simulink model "rwnn_pid_pso"  (R2021a)
settings: Solver=VariableStepAuto  StartTime=0.0  StopTime=10.0  RelTol=1e-3
PreLoadFcn:
  | b1=1
  | b2=1
  | b3=1
  | b4=1
  | a1=1
  | a2=1
  | a3=1
  | a4=1
  | qq1=1
  | qq2=1
  | qq3=1
  | qq4=1
  | w1=1
  | w2=1
  | w3=1
  | w4=1
  | ql=1
libraries: pid_lib x1
settings Model: Creator=mynam  LastModifiedBy=mynam

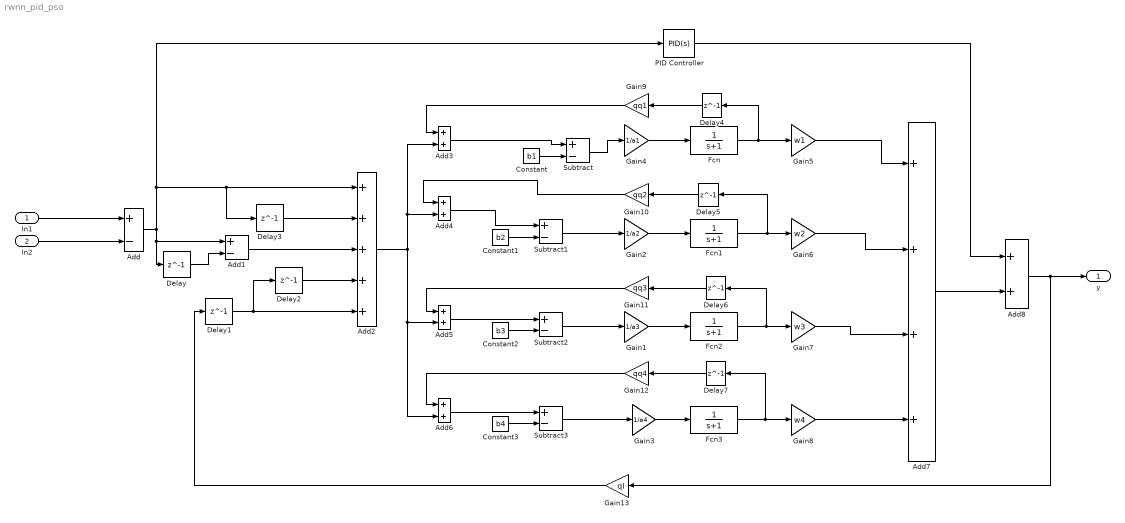
== system rwnn_pid_pso ==
  In1 : Inport
  In2 : Inport  Port=2
   Fcn{,1..3} (4 alike) : TransferFcn  Denominator=[1 1]
  Add : Sum  Inputs=+-
  Add1 : Sum  Inputs=+-
  Add2 : Sum  Inputs=+++++
  Add{3..6,8} (5 alike) : Sum
  Add7 : Sum  Inputs=++++
  Constant : Constant  Value=b1
  Constant1 : Constant  Value=b2
  Constant2 : Constant  Value=b3
  Constant3 : Constant  Value=b4
  Delay{,1..7} (8 alike) : Delay  DelayLength=1
  Gain1 : Gain  Gain=1/a3
  Gain10 : Gain  Gain=qq2
  Gain11 : Gain  Gain=qq3
  Gain12 : Gain  Gain=qq4
  Gain13 : Gain  Gain=ql
  Gain2 : Gain  Gain=1/a2
  Gain3 : Gain  Gain=1/a4
  Gain4 : Gain  Gain=1/a1
  Gain5 : Gain  Gain=w1
  Gain6 : Gain  Gain=w2
  Gain7 : Gain  Gain=w3
  Gain8 : Gain  Gain=w4
  Gain9 : Gain  Gain=qq1
  PID Controller : pid_lib/PID Controller  Controller=PID  Form=Parallel  TimeDomain=Continuous-time  UseExternalTs=off  SampleTime=-1  IntegratorMethod=Forward Euler  FilterMethod=Forward Euler  ControllerParametersSource=internal  P=1  I=1  D=0  UseFilter=on  N=100  TunerSelectOption=Transfer Function Based (PID Tuner App)  InitialConditionSource=internal  InitialConditionForIntegrator=0  InitialConditionForFilter=0  DifferentiatorICPrevScaledInput=0  ExternalReset=none  TrackingMode=off  Kt=1  LimitOutput=off  SatLimitsSource=internal  UpperSaturationLimit=inf  LowerSaturationLimit=-inf  LinearizeAsGain=on  AntiWindupMode=none  Kb=1  POutMin=[]  POutMax=[]  IOutMin=[]  IOutMax=[]  DOutMin=[]  DOutMax=[]  NOutMin=[]  NOutMax=[]  SumOutMin=[]  SumOutMax=[]  SaturationOutMin=[]  SaturationOutMax=[]  PParamMin=[]  PParamMax=[]  IParamMin=[]  IParamMax=[]  DParamMin=[]  DParamMax=[]  NParamMin=[]  NParamMax=[]  KbParamMin=[]  KbParamMax=[]  KtParamMin=[]  KtParamMax=[]  KbOutMin=[]  KbOutMax=[]  KtOutMin=[]  KtOutMax=[]  IntegratorOutMin=[]  IntegratorOutMax=[]  FilterOutMin=[]  FilterOutMax=[]  SumI1OutMin=[]  SumI1OutMax=[]  SumI2OutMin=[]  SumI2OutMax=[]  SumI3OutMin=[]  SumI3OutMax=[]  SumI4OutMin=[]  SumI4OutMax=[]  SumDOutMin=[]  SumDOutMax=[]  DifferentiatorOutMin=[]  DifferentiatorOutMax=[]  FilterDiffOutCoefMin=[]  FilterDiffOutCoefMax=[]  ReciprocalOutMin=[]  ReciprocalOutMax=[]  SumDenOutMin=[]  SumDenOutMax=[]  SumNumOutMin=[]  SumNumOutMax=[]  DivideOutMin=[]  DivideOutMax=[]  UdiffTsProdOutMin=[]  UdiffTsProdOutMax=[]  NTsProdOutMin=[]  NTsProdOutMax=[]  UintegralTsProdOutMin=[]  UintegralTsProdOutMax=[]  UngainTsProdOutMin=[]  UngainTsProdOutMax=[]  IntegratorContinuousStateAttributes=''  IntegratorStateMustResolveToSignalObject=off  IntegratorRTWStateStorageClass=Auto  FilterContinuousStateAttributes=''  FilterStateMustResolveToSignalObject=off  FilterRTWStateStorageClass=Auto  ParallelPVariant=InternalParameters  IdealPVariant=Disabled  IVariant=InternalParameters  DVariant=InternalParameters  IntegratorVariant=Continuous  SatVariant=Disabled  AWVariant=Passthrough  PCopyVariant=Disabled  TRVariant=Disabled  FdbkBlocksVariant=Forward  IdealPFdbkVariant=Disabled  SatFdbkVariant=Disabled  DerivativeFilterVariant=ContFilter  NVariant=InternalParameters  NCopyVariant=Disabled  FilterICVariant=InternalICsFilter  IntegratorICVariant=InternalICs  ExternalResetVariant=Disabled  TRSumVariant=Passthrough  SumFdbkVariant=Disabled  SumVariant=Sum_PID  TsampFilterVariant=InternalTs  TsampNgainVariant=Passthrough  TsampIntegralVariant=Passthrough  ExternalSaturationOutDataTypeStr=Inherit: Same as second input
  Subtract{,1..3} (4 alike) : Sum  Inputs=+-
  y : Outport
  wires:
  In1/1 -> Add/1
  In2/1 -> Add/2
  Delay/1 -> Add1/2
  Add/1 -> PID Controller/1, Delay3/1, Add2/1, Add1/1, Delay/1
  Delay3/1 -> Add2/2
  Add1/1 -> Add2/3
  Delay2/1 -> Add2/4
  Delay1/1 -> Delay2/1, Add2/5
  Add2/1 -> Add6/2, Add5/2, Add4/2, Add3/2
  Add3/1 -> Subtract/1
  Constant/1 -> Subtract/2
  Constant1/1 -> Subtract1/2
  Constant2/1 -> Subtract2/2
  Constant3/1 -> Subtract3/2
  Add4/1 -> Subtract1/1
  Add5/1 -> Subtract2/1
  Add6/1 -> Subtract3/1
  Subtract/1 -> Gain4/1
  Subtract1/1 -> Gain2/1
  Subtract2/1 -> Gain1/1
  Subtract3/1 -> Gain3/1
  Gain4/1 -> " Fcn"/1
  Gain2/1 -> " Fcn1"/1
  Gain1/1 -> " Fcn2"/1
  Gain3/1 -> " Fcn3"/1
  " Fcn"/1 -> Delay4/1, Gain5/1
  " Fcn1"/1 -> Delay5/1, Gain6/1
  " Fcn2"/1 -> Delay6/1, Gain7/1
  " Fcn3"/1 -> Delay7/1, Gain8/1
  Delay4/1 -> Gain9/1
  Delay5/1 -> Gain10/1
  Delay6/1 -> Gain11/1
  Delay7/1 -> Gain12/1
  Gain11/1 -> Add5/1
  Gain10/1 -> Add4/1
  Gain9/1 -> Add3/1
  Gain12/1 -> Add6/1
  Gain5/1 -> Add7/1
  Gain6/1 -> Add7/2
  Gain7/1 -> Add7/3
  Gain8/1 -> Add7/4
  Add7/1 -> Add8/2
  Add8/1 -> Gain13/1, y/1
  PID Controller/1 -> Add8/1
  Gain13/1 -> Delay1/1
